simulink model "Display"  (R2020a)
settings: Solver=VariableStepAuto  StartTime=0.0  StopTime=10.0  RelTol=1e-3
settings Model: Creator=royde  LastModifiedBy=royde

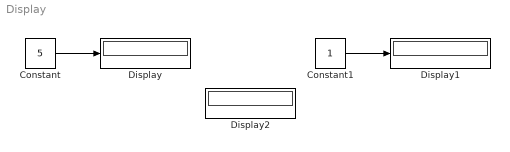
== system Display ==
  Constant : Constant  Value=5
  Constant1 : Constant
  Display : Display
  Display1 : Display
  Display2 : Display
      settings: Floating=on
  wires:
  Constant1/1 -> Display1/1
  Constant/1 -> Display/1
